simulink model "fixpt_derived_minmax"  (R2015b)
settings: Solver=FixedStepDiscrete  SolverMode=SingleTasking  StartTime=0.0  StopTime=10  RelTol=1e-3
PreLoadFcn:
  | [num,den] = butter(1,0.3);
libraries: simulink x1
settings Model: FPTRunName=FPA 参照  Creator=y_yama  LastModifiedBy=amatsumo
settings DataIOCC: SaveFormat=Array  SignalLoggingSaveFormat=ModelDataLogs  SaveOutput=off  SaveTime=off
settings OptimizationCC: BlockReduction=off  ConditionallyExecuteInputs=off  DefaultParameterBehavior=Inlined  InlineInvariantSignals=on  ExpressionDepthLimit=2147483647  ZeroExternalMemoryAtStartup=off  ZeroInternalMemoryAtStartup=off  InitFltsAndDblsToZero=on  NoFixptDivByZeroProtection=on  EfficientFloat2IntCast=on  OptimizeModelRefInitCode=on  LifeSpan=1
settings DebuggingCC: AlgebraicLoopMsg=error  UnderspecifiedInitializationDetection=Classic  MergeDetectMultiDrivingBlocksExec=none  SolverPrmCheckMsg=warning  InheritedTsInSrcMsg=none  SingleTaskRateTransMsg=error  ParameterPrecisionLossMsg=none  FcnCallInpInsideContextMsg=UseLocalSettings  StateNameClashWarn=warning
settings HardwareCC: ProdBitPerPointer=32  ProdLargestAtomicFloat=None  ProdIntDivRoundTo=Undefined  ProdEndianess=Unspecified  ProdWordSize=32  ProdHWDeviceType=ASIC/FPGA->ASIC/FPGA  TargetBitPerPointer=64  TargetLongLongMode=on  TargetIntDivRoundTo=Zero  TargetEndianess=LittleEndian  TargetWordSize=64  TargetHWDeviceType=MATLAB Host  ProdEqTarget=off
settings RTWCC: SystemTargetFile=ert.tlc  GenCodeOnly=on  TemplateMakefile=ert_default_tmf  Description=Real-Time Workshop Embedded Coder (no auto configuration)  GenerateReport=on  IncludeHyperlinkInReport=on  LaunchReport=on
settings CodeAppCC: GenerateComments=off  IgnoreCustomStorageClasses=off  CustomSymbolStrGlobalVar=$N$M  CustomSymbolStrType=$N$R$M  SimulinkBlockComments=off  InternalIdentifier=Classic
settings ERTTargetCC: GenerateSampleERTMain=on  IncludeMdlTerminateFcn=off  SuppressErrorStatus=on  SupportAbsoluteTime=off  SupportNonFinite=off  SupportComplex=off  PurelyIntegerCode=on  InlinedParameterPlacement=NonHierarchical  ERTCustomFileTemplate=example_file_process.tlc
settings ConfigComp: CovModelRefEnable=Off  CovSFcnEnable=off

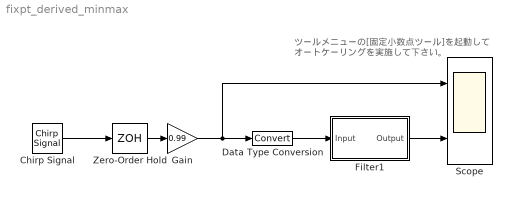
== system fixpt_derived_minmax ==
  note: ツールメニューの[固定小数点ツール]を起動して
      | オートケーリングを実施して下さい。
  Chirp Signal : simulink/Sources/Chirp Signal  f1=10  T=10  f2=500
  Data Type Conversion : DataTypeConversion
  Filter1 : Subsystem  Tag=FilterWizardSubSystem  TreatAsAtomicUnit=on  MinMaxOverflowLogging=MinMaxAndOverflow
      settings: ErrorFcn=dspFilterRealizedInBasicElemsAlgLoopErrFcnCallback
  Gain : Gain  Gain=0.99
  Scope : Scope  NumInputPorts=2
  Zero-Order Hold : ZeroOrderHold  SampleTime=1/1000
  wires:
  Zero-Order Hold/1 -> Gain/1
  Filter1/1(Output) -> Scope/2
  Chirp Signal/1 -> Zero-Order Hold/1
  Gain/1 -> Data Type Conversion/1, Scope/1
  Data Type Conversion/1 -> Filter1/1(Input)

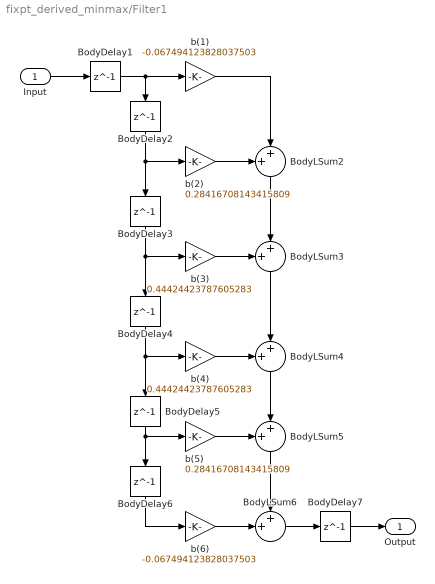
== system fixpt_derived_minmax/Filter1 ==
  Input : Inport  OutMin=-1  OutMax=1  OutDataTypeStr=double
  BodyDelay{1..7} (7 alike) : Delay  DelayLength=1  InitialCondition=0  InputProcessing=Columns as channels (frame based)
  BodyLSum{2..6} (5 alike) : Sum  Inputs=++|  OutDataTypeStr=double  RndMeth=Nearest  SaturateOnIntegerOverflow=on
  b(1) : Gain  Gain=-0.067494123828037503  ParamDataTypeStr=double  OutDataTypeStr=double  RndMeth=Nearest  SaturateOnIntegerOverflow=on
  b(2) : Gain  Gain=0.28416708143415809  ParamDataTypeStr=double  OutDataTypeStr=double  RndMeth=Nearest  SaturateOnIntegerOverflow=on
  b(3) : Gain  Gain=0.44424423787605283  ParamDataTypeStr=double  OutDataTypeStr=double  RndMeth=Nearest  SaturateOnIntegerOverflow=on
  b(4) : Gain  Gain=0.44424423787605283  ParamDataTypeStr=double  OutDataTypeStr=double  RndMeth=Nearest  SaturateOnIntegerOverflow=on
  b(5) : Gain  Gain=0.28416708143415809  ParamDataTypeStr=double  OutDataTypeStr=double  RndMeth=Nearest  SaturateOnIntegerOverflow=on
  b(6) : Gain  Gain=-0.067494123828037503  ParamDataTypeStr=double  OutDataTypeStr=double  RndMeth=Nearest  SaturateOnIntegerOverflow=on
  Output : Outport
  wires:
  Input/1 -> BodyDelay1/1
  b(1)/1 -> BodyLSum2/2
  BodyDelay2/1 -> BodyDelay3/1, b(2)/1
  b(2)/1 -> BodyLSum2/1
  BodyLSum2/1 -> BodyLSum3/2
  BodyDelay3/1 -> BodyDelay4/1, b(3)/1
  b(3)/1 -> BodyLSum3/1
  BodyLSum3/1 -> BodyLSum4/2
  BodyDelay4/1 -> BodyDelay5/1, b(4)/1
  b(4)/1 -> BodyLSum4/1
  BodyLSum4/1 -> BodyLSum5/2
  BodyDelay5/1 -> BodyDelay6/1, b(5)/1
  b(5)/1 -> BodyLSum5/1
  BodyLSum5/1 -> BodyLSum6/1
  BodyDelay6/1 -> b(6)/1
  b(6)/1 -> BodyLSum6/2
  BodyLSum6/1 -> BodyDelay7/1
  BodyDelay1/1 -> b(1)/1, BodyDelay2/1
  BodyDelay7/1 -> Output/1
